simulink model "missiontest"  (R2018a)
settings: Solver=VariableStepAuto  StartTime=0.0  StopTime=0  RelTol=1e-3
libraries: aerolibatmos2 x1
settings Model: Creator=mairon  LastModifiedBy=mairon

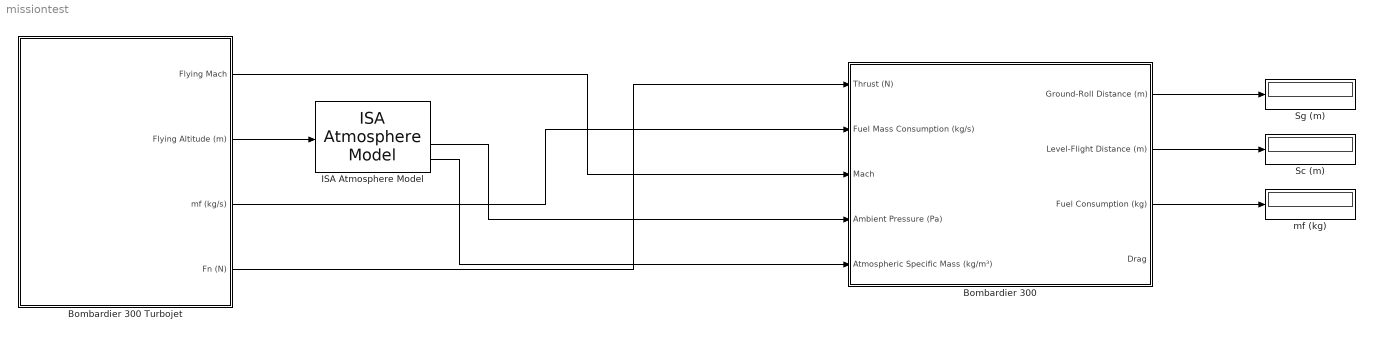
== system missiontest ==
  Bombardier 300 : Subsystem  AncestorBlock=motorlib/Concorde
  Bombardier 300 Turbojet : Subsystem  AncestorBlock=motorlib/Concorde Turbojet
  ISA Atmosphere Model : aerolibatmos2/ISA Atmosphere Model  custom=off  g=9.80665  gamma=1.4  R=287.0531  L=0.0065  h_trop=11000  h_strat=20000  rho0=1.225  P0=101325  T0=288.15  h0=0
      settings: SourceProductName=Aerospace Blockset
  Sc (m) : Display
  Sg (m) : Display
  mf (kg) : Display
  wires:
  Bombardier 300/3(Fuel Consumption (kg)) -> mf (kg)/1
  Bombardier 300/2(Level-Flight Distance (m)) -> Sc (m)/1
  Bombardier 300/1(Ground-Roll Distance (m)) -> Sg (m)/1
  Bombardier 300 Turbojet/1(Flying Mach) -> Bombardier 300/3(Mach)
  Bombardier 300 Turbojet/3(mf (kg/s)) -> Bombardier 300/2(Fuel Mass Consumption (kg/s))
  Bombardier 300 Turbojet/4(Fn (N)) -> Bombardier 300/1(Thrust (N))
  Bombardier 300 Turbojet/2(Flying Altitude (m)) -> ISA Atmosphere Model/1
  ISA Atmosphere Model/3 -> Bombardier 300/4(Ambient Pressure (Pa))
  ISA Atmosphere Model/4 -> Bombardier 300/5(Atmospheric Specific Mass (kg/m³))

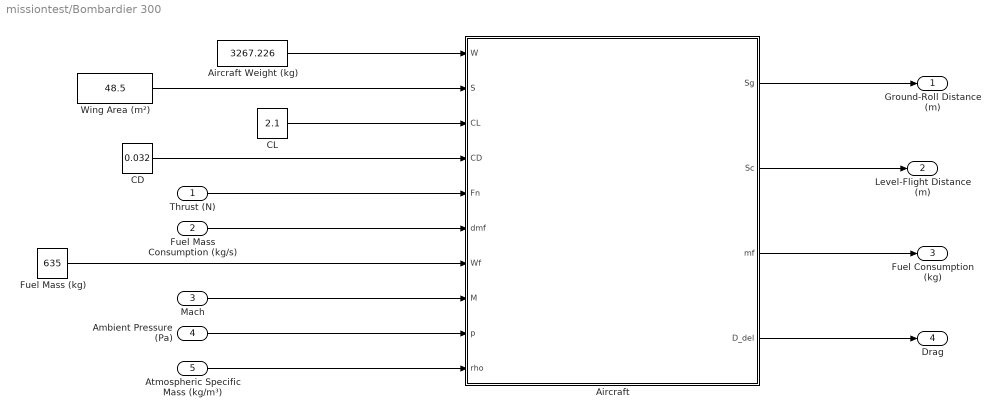
== system missiontest/Bombardier 300 ==
  Thrust (N) : Inport
  Fuel Mass Consumption (kg/s) : Inport  Port=2
  Mach : Inport  Port=3
  Ambient Pressure (Pa) : Inport  Port=4
  Atmospheric Specific Mass (kg/m³) : Inport  Port=5
  Aircraft : MATLAB Function  TreatAsAtomicUnit=on
  Aircraft Weight (kg) : Constant  Value=3267.226
  CD : Constant  Value=0.032
  CL : Constant  Value=2.1
  Fuel Mass (kg) : Constant  Value=635
  Wing Area (m²) : Constant  Value=48.5
  Ground-Roll Distance (m) : Outport
  Level-Flight Distance (m) : Outport  Port=2
  Fuel Consumption (kg) : Outport  Port=3
  Drag : Outport  Port=4
  wires:
  Aircraft/1(Sg) -> Ground-Roll Distance (m)/1
  Aircraft/2(Sc) -> Level-Flight Distance (m)/1
  Ambient Pressure (Pa)/1 -> Aircraft/9(p)
  Fuel Mass Consumption (kg/s)/1 -> Aircraft/6(dmf)
  Aircraft/3(mf) -> Fuel Consumption (kg)/1
  Mach/1 -> Aircraft/8(M)
  Thrust (N)/1 -> Aircraft/5(Fn)
  Fuel Mass (kg)/1 -> Aircraft/7(Wf)
  Atmospheric Specific Mass (kg/m³)/1 -> Aircraft/10(rho)
  Wing Area (m²)/1 -> Aircraft/2(S)
  CD/1 -> Aircraft/4(CD)
  CL/1 -> Aircraft/3(CL)
  Aircraft Weight (kg)/1 -> Aircraft/1(W)
  Aircraft/4(D_del) -> Drag/1

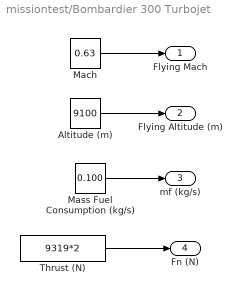
== system missiontest/Bombardier 300 Turbojet ==
  Altitude (m) : Constant  Value=9100
  Mach : Constant  Value=0.63
  Mass Fuel Consumption (kg/s) : Constant  Value=0.100
  Thrust (N) : Constant  Value=9319*2
  Flying Mach : Outport
  Flying Altitude (m) : Outport  Port=2
  mf (kg/s) : Outport  Port=3
  Fn (N) : Outport  Port=4
  wires:
  Altitude (m)/1 -> Flying Altitude (m)/1
  Mass Fuel Consumption (kg/s)/1 -> mf (kg/s)/1
  Mach/1 -> Flying Mach/1
  Thrust (N)/1 -> Fn (N)/1

== matlab function missiontest/Bombardier 300/Aircraft ==
  data: W input; Sg output; S input; CL input; CD input; Fn input; dmf input; Wf input; M input; Sc output; mf output; p input; rho input; D_del output
function [Sg,Sc,mf,D_del] = Aircraft(W,S,CL,CD,Fn,dmf,Wf,M,p,rho)
    g = 9.81;   % [m/s^2]  gravity acceleration
    mu = 0.02;  %          fricction coefficient
    p_std = 101.3e3; % [Pa] standard pressure
    gamma = 1.4;    % specific heat ratio
    
    W = (W+Wf)*g;    % [N] weight
   
    Vstall = sqrt(W/(0.5*CL*rho*S));    % [m/s] stall velocity
    Vlo = Vstall*1.2;                   % [m/s] lift-off velocity
    
    a = g*(Fn - mu*W)/W;    % [m/s^2] mean acceleration 
    Sg = Vlo^2/(2*a);       % [m] ground-roll distance
    
    dt = Vlo/(2*a)        % [s] ground-roll time
    
    t = Wf/dmf
    Sc = t*(M*340)
    mf=Wf
    
    TSFC = dmf/Fn
    Sc = M*340/g * 1/TSFC * CL/CD * log((W+Wf)/W)
    
    
    % [m] level flight distance
    %Sc = (2/(TSFC*g))*sqrt(2*CL/(S*rho*CD))*(sqrt(W)-sqrt(W-Wf))
    %t = Sc/(M*340)
    
    %mf = dmf*dt
    %mf = dmf*(dt+t)    % [kg]   fuel mass consumption per flight
   
    del = p/p_std;
    
    % power required
    M = 0:0.02:0.9;
    D_del = gamma*0.5*p_std*CL*M.^2*S;
    
    % power available
    Fn_del = Fn/del;
